simulink model "TST_ExtDem_SelectParameter"  (R2016b)
settings: Solver=FixedStepDiscrete  StartTime=0.0  StopTime=simTime  FixedStep=sampleTime  RelTol=1e-3
values from neighbouring files (symbols this model uses):
  testCase = 1    [initTST_ExtDem_SelectParameter_001.m]
libraries: simulink x34, UnitTest_Lib x32
(part 2 of 2)

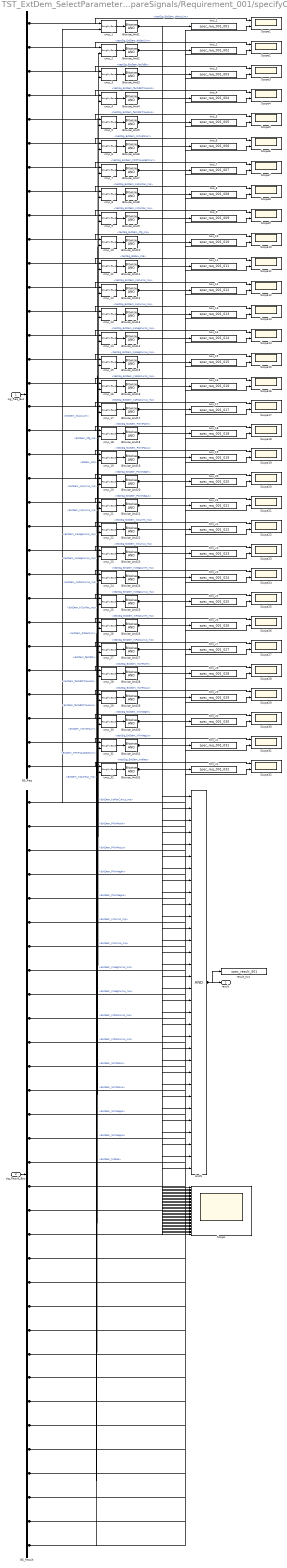
== system TST_ExtDem_SelectParameter/compareSignals/Requirement_001/specifyOutputs ==
  sig_Req_Bus : Inport
  sig_Result_Bus : Inport  Port=2
  AndN : Logic  Inputs=32
  BS_Req : BusSelector  OutputSignals=testSig_ExtDem_dnAccLim,testSig_ExtDem_dnDeclLim,testSig_ExtDem_facFdbk,testSig_ExtDem_facFdbkTrqLosHi,testSig_ExtDem_facFdbkTrqLosLo,testSig_ExtDem_InrtVehCurr,testSig_ExtDem_tiFltTrqLosEstCurr,testSig_ExtDem_KpCorFac_mp,testSig_ExtDem_KiCorFac_mp,testSig_ExtDem_Cfg_mp,testSig_EISGov_st6,testSig_ExtDem_KpCurrHi_mp,testSig_ExtDem_KpCurrLo_mp,testSig_ExtDem_KpNegCurrHi_mp,testSig_ExtDem_KpNegCurrLo_mp,testSig_ExtDem_KpPosCurrHi_mp,testSig_ExtDem_KpPosCurrLo_mp,testSig_ExtDem_PWinPosHi,testSig_ExtDem_PWinPosLo,testSig_ExtDem_PWinNegHi,testSig_ExtDem_PWinNegLo,testSig_ExtDem_KiCurrHi_mp,testSig_ExtDem_KiCurrLo_mp,testSig_ExtDem_KiNegCurrHi_mp,testSig_ExtDem_KiNegCurrLo_mp,testSig_ExtDem_KiPosCurrHi_mp,testSig_ExtDem_KiPosCurrLo_mp,testSig_ExtDem_IWinPosHi,testSig_ExtDem_IWinPosLo,testSig_ExtDem_IWinNegHi,testSig_ExtDem_IWinNegLo,testSig_ExtDem_trqReq
  BS_Result : BusSelector  OutputSignals=ExtDem_dnAccLim,ExtDem_dnDeclLim,ExtDem_facFdbk,ExtDem_facFdbkTrqLosHi,ExtDem_facFdbkTrqLosLo,ExtDem_InrtVehCurr,ExtDem_tiFltTrqLosEstCurr,ExtDem_KpCorFac_mp,ExtDem_KiCorFac_mp,ExtDem_Cfg_mp,EISGov_st6,ExtDem_KpCurrHi_mp,ExtDem_KpCurrLo_mp,ExtDem_KpNegCurrHi_mp,ExtDem_KpNegCurrLo_mp,ExtDem_KpPosCurrHi_mp,ExtDem_KpPosCurrLo_mp,ExtDem_PWinPosHi,ExtDem_PWinPosLo,ExtDem_PWinNegHi,ExtDem_PWinNegLo,ExtDem_KiCurrHi_mp,ExtDem_KiCurrLo_mp,ExtDem_KiNegCurrHi_mp,ExtDem_KiNegCurrLo_mp,ExtDem_KiPosCurrHi_mp,ExtDem_KiPosCurrLo_mp,ExtDem_IWinPosHi,ExtDem_IWinPosLo,ExtDem_IWinNegHi,ExtDem_IWinNegLo,ExtDem_trqReq
  Bitwise_And{1..32} (32 alike) : simulink/Logic and Bit Operations/Bitwise Operator  logicop=AND  UseBitMask=off  BitMask=bin2dec('11011001')  BitMaskRealWorld=Stored Integer
  Scope : Scope  NumInputPorts=32
  Scope{1..32} (32 alike) : Scope  NumInputPorts=2
  cmp_{1..32} (32 alike) : UnitTest_Lib/RoughlyEqual  slope=0.1
  result_tws : ToWorkspace  VariableName=spec_result_001
  tws_1 : ToWorkspace  VariableName=spec_req_001_001
  tws_10 : ToWorkspace  VariableName=spec_req_001_010
  tws_11 : ToWorkspace  VariableName=spec_req_001_011
  tws_12 : ToWorkspace  VariableName=spec_req_001_012
  tws_13 : ToWorkspace  VariableName=spec_req_001_013
  tws_14 : ToWorkspace  VariableName=spec_req_001_014
  tws_15 : ToWorkspace  VariableName=spec_req_001_015
  tws_16 : ToWorkspace  VariableName=spec_req_001_016
  tws_17 : ToWorkspace  VariableName=spec_req_001_017
  tws_18 : ToWorkspace  VariableName=spec_req_001_018
  tws_19 : ToWorkspace  VariableName=spec_req_001_019
  tws_2 : ToWorkspace  VariableName=spec_req_001_002
  tws_20 : ToWorkspace  VariableName=spec_req_001_020
  tws_21 : ToWorkspace  VariableName=spec_req_001_021
  tws_22 : ToWorkspace  VariableName=spec_req_001_022
  tws_23 : ToWorkspace  VariableName=spec_req_001_023
  tws_24 : ToWorkspace  VariableName=spec_req_001_024
  tws_25 : ToWorkspace  VariableName=spec_req_001_025
  tws_26 : ToWorkspace  VariableName=spec_req_001_026
  tws_27 : ToWorkspace  VariableName=spec_req_001_027
  tws_28 : ToWorkspace  VariableName=spec_req_001_028
  tws_29 : ToWorkspace  VariableName=spec_req_001_029
  tws_3 : ToWorkspace  VariableName=spec_req_001_003
  tws_30 : ToWorkspace  VariableName=spec_req_001_030
  tws_31 : ToWorkspace  VariableName=spec_req_001_031
  tws_32 : ToWorkspace  VariableName=spec_req_001_032
  tws_4 : ToWorkspace  VariableName=spec_req_001_004
  tws_5 : ToWorkspace  VariableName=spec_req_001_005
  tws_6 : ToWorkspace  VariableName=spec_req_001_006
  tws_7 : ToWorkspace  VariableName=spec_req_001_007
  tws_8 : ToWorkspace  VariableName=spec_req_001_008
  tws_9 : ToWorkspace  VariableName=spec_req_001_009
  result : Outport
  wires:
  sig_Req_Bus/1 -> BS_Req/1
  sig_Result_Bus/1 -> BS_Result/1
  AndN/1 -> result/1, result_tws/1
  BS_Req/1 -> cmp_1/1, Scope1/1  "<testSig_ExtDem_dnAccLim>"
  BS_Result/1 -> cmp_1/2, Scope1/2  "<ExtDem_dnAccLim>"
  cmp_1/1 -> Bitwise_And1/1
  Bitwise_And1/1 -> tws_1/1, AndN/1, Scope/1
  BS_Req/2 -> cmp_2/1, Scope2/1  "<testSig_ExtDem_dnDeclLim>"
  BS_Result/2 -> cmp_2/2, Scope2/2  "<ExtDem_dnDeclLim>"
  cmp_2/1 -> Bitwise_And2/1
  Bitwise_And2/1 -> tws_2/1, AndN/2, Scope/2
  BS_Req/3 -> cmp_3/1, Scope3/1  "<testSig_ExtDem_facFdbk>"
  BS_Result/3 -> cmp_3/2, Scope3/2  "<ExtDem_facFdbk>"
  cmp_3/1 -> Bitwise_And3/1
  Bitwise_And3/1 -> tws_3/1, AndN/3, Scope/3
  BS_Req/4 -> cmp_4/1, Scope4/1  "<testSig_ExtDem_facFdbkTrqLosHi>"
  BS_Result/4 -> cmp_4/2, Scope4/2  "<ExtDem_facFdbkTrqLosHi>"
  cmp_4/1 -> Bitwise_And4/1
  Bitwise_And4/1 -> tws_4/1, AndN/4, Scope/4
  BS_Req/5 -> cmp_5/1, Scope5/1  "<testSig_ExtDem_facFdbkTrqLosLo>"
  BS_Result/5 -> cmp_5/2, Scope5/2  "<ExtDem_facFdbkTrqLosLo>"
  cmp_5/1 -> Bitwise_And5/1
  Bitwise_And5/1 -> tws_5/1, AndN/5, Scope/5
  BS_Req/6 -> cmp_6/1, Scope6/1  "<testSig_ExtDem_InrtVehCurr>"
  BS_Result/6 -> cmp_6/2, Scope6/2  "<ExtDem_InrtVehCurr>"
  cmp_6/1 -> Bitwise_And6/1
  Bitwise_And6/1 -> tws_6/1, AndN/6, Scope/6
  BS_Req/7 -> cmp_7/1, Scope7/1  "<testSig_ExtDem_tiFltTrqLosEstCurr>"
  BS_Result/7 -> cmp_7/2, Scope7/2  "<ExtDem_tiFltTrqLosEstCurr>"
  cmp_7/1 -> Bitwise_And7/1
  Bitwise_And7/1 -> tws_7/1, AndN/7, Scope/7
  BS_Req/8 -> cmp_8/1, Scope8/1  "<testSig_ExtDem_KpCorFac_mp>"
  BS_Result/8 -> cmp_8/2, Scope8/2  "<ExtDem_KpCorFac_mp>"
  cmp_8/1 -> Bitwise_And8/1
  Bitwise_And8/1 -> tws_8/1, AndN/8, Scope/8
  BS_Req/9 -> cmp_9/1, Scope9/1  "<testSig_ExtDem_KiCorFac_mp>"
  BS_Result/9 -> cmp_9/2, Scope9/2  "<ExtDem_KiCorFac_mp>"
  cmp_9/1 -> Bitwise_And9/1
  Bitwise_And9/1 -> tws_9/1, AndN/9, Scope/9
  BS_Req/10 -> cmp_10/1, Scope10/1  "<testSig_ExtDem_Cfg_mp>"
  BS_Result/10 -> cmp_10/2, Scope10/2  "<ExtDem_Cfg_mp>"
  cmp_10/1 -> Bitwise_And10/1
  Bitwise_And10/1 -> tws_10/1, AndN/10, Scope/10
  BS_Req/11 -> cmp_11/1, Scope11/1  "<testSig_EISGov_st6>"
  BS_Result/11 -> cmp_11/2, Scope11/2  "<EISGov_st6>"
  cmp_11/1 -> Bitwise_And11/1
  Bitwise_And11/1 -> tws_11/1, AndN/11, Scope/11
  BS_Req/12 -> cmp_12/1, Scope12/1  "<testSig_ExtDem_KpCurrHi_mp>"
  BS_Result/12 -> cmp_12/2, Scope12/2  "<ExtDem_KpCurrHi_mp>"
  cmp_12/1 -> Bitwise_And12/1
  Bitwise_And12/1 -> tws_12/1, AndN/12, Scope/12
  BS_Req/13 -> cmp_13/1, Scope13/1  "<testSig_ExtDem_KpCurrLo_mp>"
  BS_Result/13 -> cmp_13/2, Scope13/2  "<ExtDem_KpCurrLo_mp>"
  cmp_13/1 -> Bitwise_And13/1
  Bitwise_And13/1 -> tws_13/1, AndN/13, Scope/13
  BS_Req/14 -> cmp_14/1, Scope14/1  "<testSig_ExtDem_KpNegCurrHi_mp>"
  BS_Result/14 -> cmp_14/2, Scope14/2  "<ExtDem_KpNegCurrHi_mp>"
  cmp_14/1 -> Bitwise_And14/1
  Bitwise_And14/1 -> tws_14/1, AndN/14, Scope/14
  BS_Req/15 -> cmp_15/1, Scope15/1  "<testSig_ExtDem_KpNegCurrLo_mp>"
  BS_Result/15 -> cmp_15/2, Scope15/2  "<ExtDem_KpNegCurrLo_mp>"
  cmp_15/1 -> Bitwise_And15/1
  Bitwise_And15/1 -> tws_15/1, AndN/15, Scope/15
  BS_Req/16 -> cmp_16/1, Scope16/1  "<testSig_ExtDem_KpPosCurrHi_mp>"
  BS_Result/16 -> cmp_16/2, Scope16/2  "<ExtDem_KpPosCurrHi_mp>"
  cmp_16/1 -> Bitwise_And16/1
  Bitwise_And16/1 -> tws_16/1, AndN/16, Scope/16
  BS_Req/17 -> cmp_17/1, Scope17/1  "<testSig_ExtDem_KpPosCurrLo_mp>"
  BS_Result/17 -> cmp_17/2, Scope17/2  "<ExtDem_KpPosCurrLo_mp>"
  cmp_17/1 -> Bitwise_And17/1
  Bitwise_And17/1 -> tws_17/1, AndN/17, Scope/17
  BS_Req/18 -> cmp_18/1, Scope18/1  "<testSig_ExtDem_PWinPosHi>"
  BS_Result/18 -> cmp_18/2, Scope18/2  "<ExtDem_PWinPosHi>"
  cmp_18/1 -> Bitwise_And18/1
  Bitwise_And18/1 -> tws_18/1, AndN/18, Scope/18
  BS_Req/19 -> cmp_19/1, Scope19/1  "<testSig_ExtDem_PWinPosLo>"
  BS_Result/19 -> cmp_19/2, Scope19/2  "<ExtDem_PWinPosLo>"
  cmp_19/1 -> Bitwise_And19/1
  Bitwise_And19/1 -> tws_19/1, AndN/19, Scope/19
  BS_Req/20 -> cmp_20/1, Scope20/1  "<testSig_ExtDem_PWinNegHi>"
  BS_Result/20 -> cmp_20/2, Scope20/2  "<ExtDem_PWinNegHi>"
  cmp_20/1 -> Bitwise_And20/1
  Bitwise_And20/1 -> tws_20/1, AndN/20, Scope/20
  BS_Req/21 -> cmp_21/1, Scope21/1  "<testSig_ExtDem_PWinNegLo>"
  BS_Result/21 -> cmp_21/2, Scope21/2  "<ExtDem_PWinNegLo>"
  cmp_21/1 -> Bitwise_And21/1
  Bitwise_And21/1 -> tws_21/1, AndN/21, Scope/21
  BS_Req/22 -> cmp_22/1, Scope22/1  "<testSig_ExtDem_KiCurrHi_mp>"
  BS_Result/22 -> cmp_22/2, Scope22/2  "<ExtDem_KiCurrHi_mp>"
  cmp_22/1 -> Bitwise_And22/1
  Bitwise_And22/1 -> tws_22/1, AndN/22, Scope/22
  BS_Req/23 -> cmp_23/1, Scope23/1  "<testSig_ExtDem_KiCurrLo_mp>"
  BS_Result/23 -> cmp_23/2, Scope23/2  "<ExtDem_KiCurrLo_mp>"
  cmp_23/1 -> Bitwise_And23/1
  Bitwise_And23/1 -> tws_23/1, AndN/23, Scope/23
  BS_Req/24 -> cmp_24/1, Scope24/1  "<testSig_ExtDem_KiNegCurrHi_mp>"
  BS_Result/24 -> cmp_24/2, Scope24/2  "<ExtDem_KiNegCurrHi_mp>"
  cmp_24/1 -> Bitwise_And24/1
  Bitwise_And24/1 -> tws_24/1, AndN/24, Scope/24
  BS_Req/25 -> cmp_25/1, Scope25/1  "<testSig_ExtDem_KiNegCurrLo_mp>"
  BS_Result/25 -> cmp_25/2, Scope25/2  "<ExtDem_KiNegCurrLo_mp>"
  cmp_25/1 -> Bitwise_And25/1
  Bitwise_And25/1 -> tws_25/1, AndN/25, Scope/25
  BS_Req/26 -> cmp_26/1, Scope26/1  "<testSig_ExtDem_KiPosCurrHi_mp>"
  BS_Result/26 -> cmp_26/2, Scope26/2  "<ExtDem_KiPosCurrHi_mp>"
  cmp_26/1 -> Bitwise_And26/1
  Bitwise_And26/1 -> tws_26/1, AndN/26, Scope/26
  BS_Req/27 -> cmp_27/1, Scope27/1  "<testSig_ExtDem_KiPosCurrLo_mp>"
  BS_Result/27 -> cmp_27/2, Scope27/2  "<ExtDem_KiPosCurrLo_mp>"
  cmp_27/1 -> Bitwise_And27/1
  Bitwise_And27/1 -> tws_27/1, AndN/27, Scope/27
  BS_Req/28 -> cmp_28/1, Scope28/1  "<testSig_ExtDem_IWinPosHi>"
  BS_Result/28 -> cmp_28/2, Scope28/2  "<ExtDem_IWinPosHi>"
  cmp_28/1 -> Bitwise_And28/1
  Bitwise_And28/1 -> tws_28/1, AndN/28, Scope/28
  BS_Req/29 -> cmp_29/1, Scope29/1  "<testSig_ExtDem_IWinPosLo>"
  BS_Result/29 -> cmp_29/2, Scope29/2  "<ExtDem_IWinPosLo>"
  cmp_29/1 -> Bitwise_And29/1
  Bitwise_And29/1 -> tws_29/1, AndN/29, Scope/29
  BS_Req/30 -> cmp_30/1, Scope30/1  "<testSig_ExtDem_IWinNegHi>"
  BS_Result/30 -> cmp_30/2, Scope30/2  "<ExtDem_IWinNegHi>"
  cmp_30/1 -> Bitwise_And30/1
  Bitwise_And30/1 -> tws_30/1, AndN/30, Scope/30
  BS_Req/31 -> cmp_31/1, Scope31/1  "<testSig_ExtDem_IWinNegLo>"
  BS_Result/31 -> cmp_31/2, Scope31/2  "<ExtDem_IWinNegLo>"
  cmp_31/1 -> Bitwise_And31/1
  Bitwise_And31/1 -> tws_31/1, AndN/31, Scope/31
  BS_Req/32 -> cmp_32/1, Scope32/1  "<testSig_ExtDem_trqReq>"
  BS_Result/32 -> cmp_32/2, Scope32/2  "<ExtDem_trqReq>"
  cmp_32/1 -> Bitwise_And32/1
  Bitwise_And32/1 -> tws_32/1, AndN/32, Scope/32
